simulink model "fxpdemo_preconvert"  (Simulink 7.6)
settings: Solver=FixedStepDiscrete  SolverMode=SingleTasking  StartTime=0.0  StopTime=200.0  FixedStep=1  RelTol=1e-3
settings Model: MinMaxOverflowLogging=ForceOff  Creator=The MathWorks Inc.  ExtModeTrigMode=oneshot  ExtModeArmWhenConnect=off  ExtModeAutoUpdateStatusClock=off
settings DataIOCC: LimitDataPoints=off  SignalLoggingName=sigsOut
settings OptimizationCC: BooleanDataType=off  InlineInvariantSignals=on
settings DebuggingCC: SaveWithParameterizedLinksMsg=none  SignalResolutionControl=TryResolveAllWithWarning  SolverPrmCheckMsg=none  MultiTaskDSMMsg=warning  MultiTaskCondExecSysMsg=none  IntegerOverflowMsg=none  ParameterDowncastMsg=warning  ParameterOverflowMsg=warning  ParameterPrecisionLossMsg=none  StrictBusMsg=None
settings HardwareCC: TargetUnknown=on
settings RTWCC: IncludeERTFirstTime=on

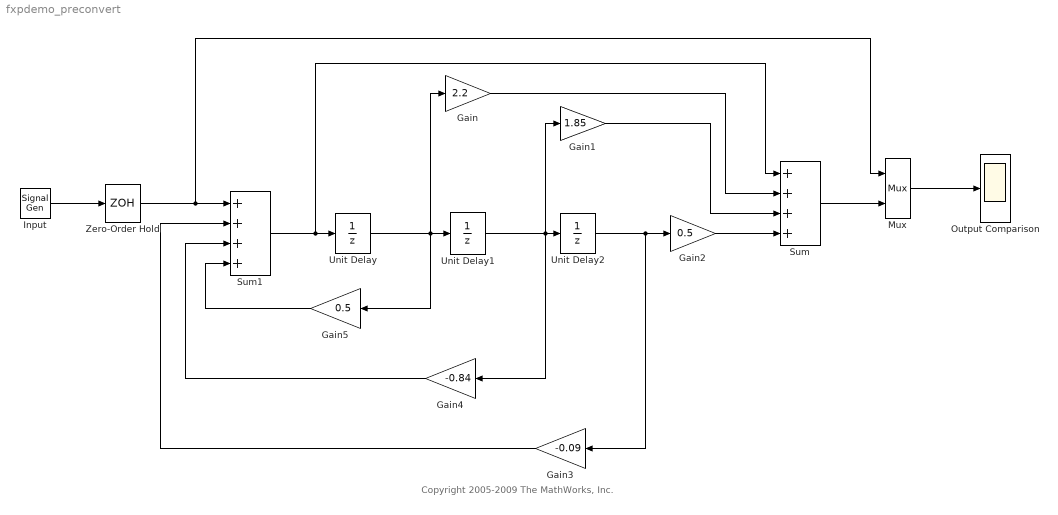
== system fxpdemo_preconvert ==
  note: Copyright 2005-2009 The MathWorks, Inc.
  Gain : Gain  Gain=2.2  SaturateOnIntegerOverflow=on  OutDataTypeStr=Inherit: Same as input  ParamDataTypeStr=Inherit: Same as input
  Gain1 : Gain  Gain=1.85  SaturateOnIntegerOverflow=on  OutDataTypeStr=Inherit: Same as input  ParamDataTypeStr=Inherit: Same as input
  Gain2 : Gain  Gain=0.5  SaturateOnIntegerOverflow=on  OutDataTypeStr=Inherit: Same as input  ParamDataTypeStr=Inherit: Same as input
  Gain3 : Gain  Gain=-0.09  SaturateOnIntegerOverflow=on  OutDataTypeStr=Inherit: Same as input  ParamDataTypeStr=Inherit: Same as input
  Gain4 : Gain  Gain=-0.84  SaturateOnIntegerOverflow=on  OutDataTypeStr=Inherit: Same as input  ParamDataTypeStr=Inherit: Same as input
  Gain5 : Gain  Gain=0.5  SaturateOnIntegerOverflow=on  OutDataTypeStr=Inherit: Same as input  ParamDataTypeStr=Inherit: Same as input
  Input : SignalGenerator  WaveForm=square  Frequency=0.005
  Mux : Mux  Inputs=2
  Output Comparison : Scope
      settings: TickLabels=on  TimeRange=200  YMin=-8  YMax=10  SaveName=OutputComparison
  Sum : Sum  Inputs=4  SaturateOnIntegerOverflow=on  InputSameDT=on  OutDataTypeStr=Inherit: Same as first input
  Sum1 : Sum  Inputs=4  SaturateOnIntegerOverflow=on  InputSameDT=on  OutDataTypeStr=Inherit: Same as first input
  Unit Delay : UnitDelay
  Unit Delay1 : UnitDelay
  Unit Delay2 : UnitDelay
  Zero-Order Hold : ZeroOrderHold
  wires:
  Input/1 -> Zero-Order Hold/1
  Sum1/1 -> Unit Delay/1, Sum/1
  Gain5/1 -> Sum1/4
  Unit Delay/1 -> Unit Delay1/1, Gain5/1, Gain/1
  Gain4/1 -> Sum1/3
  Unit Delay1/1 -> Unit Delay2/1, Gain4/1, Gain1/1
  Gain3/1 -> Sum1/2
  Gain2/1 -> Sum/4
  Gain1/1 -> Sum/3
  Gain/1 -> Sum/2
  Unit Delay2/1 -> Gain2/1, Gain3/1
  Zero-Order Hold/1 -> Sum1/1, Mux/1
  Sum/1 -> Mux/2
  Mux/1 -> Output Comparison/1
